simulink model "hpt_dual_hpt_sac"  (R2025a)
settings: Solver=ode23tb  StartTime=0.0  StopTime=0.6  RelTol=1e-3
libraries: spsLinearTransformerLib x6, spsThreePhaseVIMeasurementLib x4, spsUniversalBridgeLib x4, spsSeriesRLCBranchLib x3, spsThreePhaseSeriesRLCLoadLib x2, spsThreePhaseSeriesRLCBranchLib x2, spsVoltageMeasurementLib x2, spsThreePhaseSourceLib x2, spsGroundLib x1, spsCurrentMeasurementLib x1, spspowerguiLib x1
settings Model: Creator=m1391  LastModifiedBy=m1391

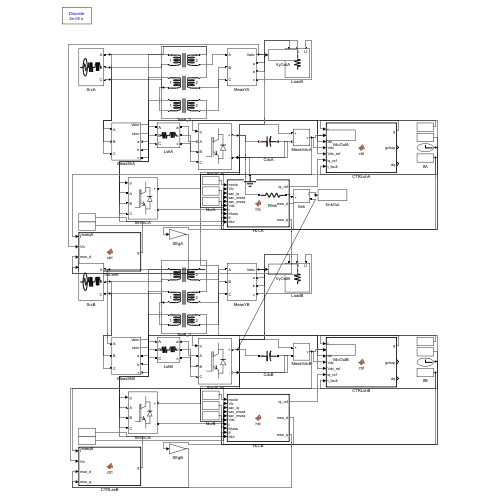
[thumbnail: Simulink's stored preview of the top-level diagram]
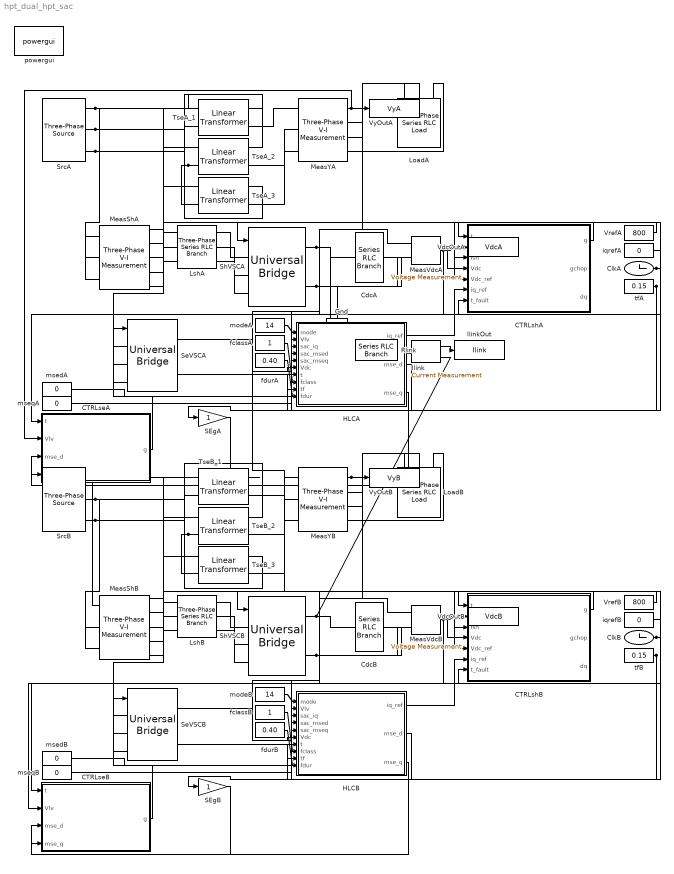
== system hpt_dual_hpt_sac ==
  CTRLseA : MATLAB Function  TreatAsAtomicUnit=on
  CTRLseB : MATLAB Function  TreatAsAtomicUnit=on
  CTRLshA : MATLAB Function  TreatAsAtomicUnit=on
  CTRLshB : MATLAB Function  TreatAsAtomicUnit=on
  CdcA : spsSeriesRLCBranchLib/Series RLC Branch  LConnTagsString=__new0  RConnTagsString=__new0  BranchType=C  Resistance=1  Inductance=1e-3  SetiL0=off  InitialCurrent=0  Capacitance=0.0022  Setx0=on  InitialVoltage=800  Measurements=None
  CdcB : spsSeriesRLCBranchLib/Series RLC Branch  LConnTagsString=__new0  RConnTagsString=__new0  BranchType=C  Resistance=1  Inductance=1e-3  SetiL0=off  InitialCurrent=0  Capacitance=0.0022  Setx0=on  InitialVoltage=800  Measurements=None
  ClkA : Clock
  ClkB : Clock
  Gnd : spsGroundLib/Ground  LConnTagsString=a
  HLCA : MATLAB Function  TreatAsAtomicUnit=on
  HLCB : MATLAB Function  TreatAsAtomicUnit=on
  Ilink : spsCurrentMeasurementLib/Current Measurement  PhasorSimulation=off  OutputType=Complex  PSBequivalent=0
  IlinkOut : ToWorkspace  VariableName=Ilink  SampleTime=2e-05
  LoadA : spsThreePhaseSeriesRLCLoadLib/Three-Phase Series RLC Load  LConnTagsString=A|B|C  Configuration=Y (floating)  NominalVoltage=400  Vabc=[1e3 1e3 1e3]  Vabcp=[1e3 1e3 1e3]  NominalFrequency=50  UnbalancedPower=off  ActivePower=400000  InductivePower=0  CapacitivePower=0  Pabc=[10e3 9e3 11e3]  QLabc=[100 90 110]  QCabc=[100 90 110]  Pabcp=[10e3 9e3 11e3]  QLabcp=[100 90 110]  QCabcp=[100 90 110]  Measurements=None  LoadType=constant Z
  LoadB : spsThreePhaseSeriesRLCLoadLib/Three-Phase Series RLC Load  LConnTagsString=A|B|C  Configuration=Y (floating)  NominalVoltage=400  Vabc=[1e3 1e3 1e3]  Vabcp=[1e3 1e3 1e3]  NominalFrequency=50  UnbalancedPower=off  ActivePower=400000  InductivePower=0  CapacitivePower=0  Pabc=[10e3 9e3 11e3]  QLabc=[100 90 110]  QCabc=[100 90 110]  Pabcp=[10e3 9e3 11e3]  QLabcp=[100 90 110]  QCabcp=[100 90 110]  Measurements=None  LoadType=constant Z
  LshA : spsThreePhaseSeriesRLCBranchLib/Three-Phase Series RLC Branch  LConnTagsString=A|B|C  RConnTagsString=A|B|C  BranchType=RL  Resistance=0.05  Inductance=0.003  Capacitance=1e-6  Measurements=None
  LshB : spsThreePhaseSeriesRLCBranchLib/Three-Phase Series RLC Branch  LConnTagsString=A|B|C  RConnTagsString=A|B|C  BranchType=RL  Resistance=0.05  Inductance=0.003  Capacitance=1e-6  Measurements=None
  MeasShA : spsThreePhaseVIMeasurementLib/Three-Phase V-I Measurement  VoltageMeasurement=phase-to-ground  SetLabelV=off  LabelV=Vabc  Vpu=off  VpuLL=off  CurrentMeasurement=yes  SetLabelI=off  LabelI=Iabc  Ipu=off  Pbase=100e6  Vbase=500e3  OutputType=Complex  PhasorSimulation=off  PSBequivalent=0
  MeasShB : spsThreePhaseVIMeasurementLib/Three-Phase V-I Measurement  VoltageMeasurement=phase-to-ground  SetLabelV=off  LabelV=Vabc  Vpu=off  VpuLL=off  CurrentMeasurement=yes  SetLabelI=off  LabelI=Iabc  Ipu=off  Pbase=100e6  Vbase=500e3  OutputType=Complex  PhasorSimulation=off  PSBequivalent=0
  MeasVdcA : spsVoltageMeasurementLib/Voltage Measurement  PhasorSimulation=off  OutputType=Complex  PSBequivalent=0
  MeasVdcB : spsVoltageMeasurementLib/Voltage Measurement  PhasorSimulation=off  OutputType=Complex  PSBequivalent=0
  MeasYA : spsThreePhaseVIMeasurementLib/Three-Phase V-I Measurement  VoltageMeasurement=phase-to-ground  SetLabelV=off  LabelV=Vabc  Vpu=off  VpuLL=off  CurrentMeasurement=no  SetLabelI=off  LabelI=Iabc  Ipu=off  Pbase=100e6  Vbase=500e3  OutputType=Complex  PhasorSimulation=off  PSBequivalent=0
  MeasYB : spsThreePhaseVIMeasurementLib/Three-Phase V-I Measurement  VoltageMeasurement=phase-to-ground  SetLabelV=off  LabelV=Vabc  Vpu=off  VpuLL=off  CurrentMeasurement=no  SetLabelI=off  LabelI=Iabc  Ipu=off  Pbase=100e6  Vbase=500e3  OutputType=Complex  PhasorSimulation=off  PSBequivalent=0
  Rlink : spsSeriesRLCBranchLib/Series RLC Branch  LConnTagsString=__new0  RConnTagsString=__new0  BranchType=R  Resistance=0.5  Inductance=1e-3  SetiL0=off  InitialCurrent=0  Capacitance=1e-6  Setx0=off  InitialVoltage=0  Measurements=None
  SEgA : Gain
  SEgB : Gain
  SeVSCA : spsUniversalBridgeLib/Universal Bridge  Arms=3  SnubberResistance=1e5  SnubberCapacitance=inf  Device=IGBT / Diodes  Ron=1e-3  Lon=0  ForwardVoltages="[  0  0  ]"  ForwardVoltage=0  GTOparameters=[ 10e-6 , 20e-6 ]  IGBTparameters=[ 1e-6 , 2e-6 ]  Measurements=None  Measurements_2=None  converterType=Rectifier
  SeVSCB : spsUniversalBridgeLib/Universal Bridge  Arms=3  SnubberResistance=1e5  SnubberCapacitance=inf  Device=IGBT / Diodes  Ron=1e-3  Lon=0  ForwardVoltages="[  0  0  ]"  ForwardVoltage=0  GTOparameters=[ 10e-6 , 20e-6 ]  IGBTparameters=[ 1e-6 , 2e-6 ]  Measurements=None  Measurements_2=None  converterType=Rectifier
  ShVSCA : spsUniversalBridgeLib/Universal Bridge  Arms=3  SnubberResistance=1e5  SnubberCapacitance=inf  Device=IGBT / Diodes  Ron=1e-3  Lon=0  ForwardVoltages="[  0  0  ]"  ForwardVoltage=0  GTOparameters=[ 10e-6 , 20e-6 ]  IGBTparameters=[ 1e-6 , 2e-6 ]  Measurements=None  Measurements_2=None  converterType=Rectifier
  ShVSCB : spsUniversalBridgeLib/Universal Bridge  Arms=3  SnubberResistance=1e5  SnubberCapacitance=inf  Device=IGBT / Diodes  Ron=1e-3  Lon=0  ForwardVoltages="[  0  0  ]"  ForwardVoltage=0  GTOparameters=[ 10e-6 , 20e-6 ]  IGBTparameters=[ 1e-6 , 2e-6 ]  Measurements=None  Measurements_2=None  converterType=Rectifier
  SrcA : spsThreePhaseSourceLib/Three-Phase Source  InternalConnection=Y  VoltagePhases=off  Voltage=400  PhaseAngle=0  Voltage_phases=[25e3 25e3 25e3]/sqrt(3)  PhaseAngles_phases=[0 -120 +120]  Frequency=50  NonIdealSource=on  SpecifyImpedance=off  Resistance=1e-3  Inductance=1e-5  ShortCircuitLevel=100e6  BaseVoltage=25e3  XRratio=7  BusType=swing  Pref=10e3  Qref=0  Prefabc=[10e3, 10e3, 10e3]  Qrefabc=[0, 0, 0]  Qmin=-inf  Qmax=inf
  SrcB : spsThreePhaseSourceLib/Three-Phase Source  InternalConnection=Y  VoltagePhases=off  Voltage=400  PhaseAngle=0  Voltage_phases=[25e3 25e3 25e3]/sqrt(3)  PhaseAngles_phases=[0 -120 +120]  Frequency=50  NonIdealSource=on  SpecifyImpedance=off  Resistance=1e-3  Inductance=1e-5  ShortCircuitLevel=100e6  BaseVoltage=25e3  XRratio=7  BusType=swing  Pref=10e3  Qref=0  Prefabc=[10e3, 10e3, 10e3]  Qrefabc=[0, 0, 0]  Qmin=-inf  Qmax=inf
  TseA_1 : spsLinearTransformerLib/Linear Transformer  UNITS=pu  NominalPower=[30000,50]  winding1=[400,0.002,0.03]  winding2=[46.2,0.002,0.03]  ThreeWindings=off  winding3=[ 315e3 0.002 0.08 ]  RmLm=[ 500 500 ]  Measurements=None  DataType=off
  TseA_2 : spsLinearTransformerLib/Linear Transformer  UNITS=pu  NominalPower=[30000,50]  winding1=[400,0.002,0.03]  winding2=[46.2,0.002,0.03]  ThreeWindings=off  winding3=[ 315e3 0.002 0.08 ]  RmLm=[ 500 500 ]  Measurements=None  DataType=off
  TseA_3 : spsLinearTransformerLib/Linear Transformer  UNITS=pu  NominalPower=[30000,50]  winding1=[400,0.002,0.03]  winding2=[46.2,0.002,0.03]  ThreeWindings=off  winding3=[ 315e3 0.002 0.08 ]  RmLm=[ 500 500 ]  Measurements=None  DataType=off
  TseB_1 : spsLinearTransformerLib/Linear Transformer  UNITS=pu  NominalPower=[30000,50]  winding1=[400,0.002,0.03]  winding2=[46.2,0.002,0.03]  ThreeWindings=off  winding3=[ 315e3 0.002 0.08 ]  RmLm=[ 500 500 ]  Measurements=None  DataType=off
  TseB_2 : spsLinearTransformerLib/Linear Transformer  UNITS=pu  NominalPower=[30000,50]  winding1=[400,0.002,0.03]  winding2=[46.2,0.002,0.03]  ThreeWindings=off  winding3=[ 315e3 0.002 0.08 ]  RmLm=[ 500 500 ]  Measurements=None  DataType=off
  TseB_3 : spsLinearTransformerLib/Linear Transformer  UNITS=pu  NominalPower=[30000,50]  winding1=[400,0.002,0.03]  winding2=[46.2,0.002,0.03]  ThreeWindings=off  winding3=[ 315e3 0.002 0.08 ]  RmLm=[ 500 500 ]  Measurements=None  DataType=off
  VdcOutA : ToWorkspace  VariableName=VdcA  SampleTime=2e-05
  VdcOutB : ToWorkspace  VariableName=VdcB  SampleTime=2e-05
  VrefA : Constant  Value=800
  VrefB : Constant  Value=800
  VyOutA : ToWorkspace  VariableName=VyA  SampleTime=2e-05
  VyOutB : ToWorkspace  VariableName=VyB  SampleTime=2e-05
  fclassA : Constant
  fclassB : Constant
  fdurA : Constant  Value=0.40
  fdurB : Constant  Value=0.40
  iqrefA : Constant  Value=0
  iqrefB : Constant  Value=0
  modeA : Constant  Value=14
  modeB : Constant  Value=14
  msedA : Constant  Value=0
  msedB : Constant  Value=0
  mseqA : Constant  Value=0
  mseqB : Constant  Value=0
  powergui : spspowerguiLib/powergui  Priority=1  SimulationMode=Discrete  SampleTime=2e-05  frequency=60  Iterations=50  frequencyindice=60  Pbase=100e6  ErrMax=1e-4  UnitsV=kV  UnitsW=MW  buscounter=0  FunctionMessages=off  echomessages=off  EnableUseOfTLC=off  CurrentSourceSwitches=off  DisableSnubberDevices=off  DisableRonSwitches=off  DisableVfSwitches=off  DisplayEquations=off  AutomaticDiscreteSolvers=off  SolverType=Tustin/Backward Euler (TBE)  Interpol=off  ExternalGateDelay=off  methode=off  Ts=100  x0status=blocks  SPID=on  SwTol=0  HookPort=off  NonlinearTolerance=1e-4  nMaxIteration=100  ContinueOnMaxIteration=off  RestoreLinks=warning  ResistiveCurrentMeasurement=off  Frange=[0:2:500]  Ylog=off  Xlog=on  ShowGrid=off  save=off  variable=ZData  structure=0  ZoomFFT=off  StartTime=0.0  cycles=1  DisplayStyle=1  fundamental=60  FreqAxis=off  MaxFrequency=1000  frequencyindicesteady=1  RmsSteady=1  display=off
  tfA : Constant  Value=0.15
  tfB : Constant  Value=0.15
  wires:
  ClkA/1 -> CTRLshA/1(t), CTRLseA/1(t), HLCA/7(t)
  MeasShA/1 -> CTRLshA/2(Vabc)
  MeasShA/2 -> CTRLshA/3(Ish)
  MeasVdcA/1 -> CTRLshA/4(Vdc), HLCA/6(Vdc), VdcOutA/1
  VrefA/1 -> CTRLshA/5(Vdc_ref)
  tfA/1 -> CTRLshA/7(t_fault), HLCA/9(tf)
  CTRLshA/1(g) -> ShVSCA/1
  MeasYA/1 -> CTRLseA/2(Vlv), HLCA/2(Vlv), VyOutA/1
  CTRLseA/1(g) -> SeVSCA/1
  modeA/1 -> HLCA/1(mode)
  iqrefA/1 -> HLCA/3(sac_iq)
  msedA/1 -> HLCA/4(sac_msed)
  mseqA/1 -> HLCA/5(sac_mseq)
  fclassA/1 -> HLCA/8(fclass)
  fdurA/1 -> HLCA/10(fdur)
  HLCA/1(iq_ref) -> CTRLshA/6(iq_ref)
  HLCA/2(mse_d) -> SEgA/1
  SEgA/1 -> CTRLseA/3(mse_d)
  HLCA/3(mse_q) -> CTRLseA/4(mse_q)
  ClkB/1 -> CTRLshB/1(t), CTRLseB/1(t), HLCB/7(t)
  MeasShB/1 -> CTRLshB/2(Vabc)
  MeasShB/2 -> CTRLshB/3(Ish)
  MeasVdcB/1 -> CTRLshB/4(Vdc), HLCB/6(Vdc), VdcOutB/1
  VrefB/1 -> CTRLshB/5(Vdc_ref)
  tfB/1 -> CTRLshB/7(t_fault), HLCB/9(tf)
  CTRLshB/1(g) -> ShVSCB/1
  MeasYB/1 -> CTRLseB/2(Vlv), HLCB/2(Vlv), VyOutB/1
  CTRLseB/1(g) -> SeVSCB/1
  modeB/1 -> HLCB/1(mode)
  iqrefB/1 -> HLCB/3(sac_iq)
  msedB/1 -> HLCB/4(sac_msed)
  mseqB/1 -> HLCB/5(sac_mseq)
  fclassB/1 -> HLCB/8(fclass)
  fdurB/1 -> HLCB/10(fdur)
  HLCB/1(iq_ref) -> CTRLshB/6(iq_ref)
  HLCB/2(mse_d) -> SEgB/1
  SEgB/1 -> CTRLseB/3(mse_d)
  HLCB/3(mse_q) -> CTRLseB/4(mse_q)
  Ilink/1 -> IlinkOut/1
  connections:
  TseA_1/RConn1 -- SrcA/RConn1 -- MeasShA/LConn1
  TseA_1/RConn2 -- MeasYA/LConn1
  MeasYA/RConn1 -- LoadA/LConn1
  MeasShA/RConn1 -- LshA/LConn1
  LshA/RConn1 -- ShVSCA/LConn1
  SeVSCA/LConn1 -- TseA_1/LConn1
  TseA_2/RConn1 -- SrcA/RConn2 -- MeasShA/LConn2
  TseA_2/RConn2 -- MeasYA/LConn2
  MeasYA/RConn2 -- LoadA/LConn2
  MeasShA/RConn2 -- LshA/LConn2
  LshA/RConn2 -- ShVSCA/LConn2
  SeVSCA/LConn2 -- TseA_2/LConn1
  TseA_3/RConn1 -- SrcA/RConn3 -- MeasShA/LConn3
  TseA_3/RConn2 -- MeasYA/LConn3
  MeasYA/RConn3 -- LoadA/LConn3
  MeasShA/RConn3 -- LshA/LConn3
  LshA/RConn3 -- ShVSCA/LConn3
  SeVSCA/LConn3 -- TseA_3/LConn1
  TseA_2/LConn2 -- TseA_1/LConn2 -- TseA_3/LConn2
  CdcA/LConn1 -- ShVSCA/RConn1 -- SeVSCA/RConn1 -- MeasVdcA/LConn1 -- Rlink/LConn1
  TseB_1/RConn1 -- SrcB/RConn1 -- MeasShB/LConn1
  TseB_1/RConn2 -- MeasYB/LConn1
  MeasYB/RConn1 -- LoadB/LConn1
  MeasShB/RConn1 -- LshB/LConn1
  LshB/RConn1 -- ShVSCB/LConn1
  SeVSCB/LConn1 -- TseB_1/LConn1
  TseB_2/RConn1 -- SrcB/RConn2 -- MeasShB/LConn2
  TseB_2/RConn2 -- MeasYB/LConn2
  MeasYB/RConn2 -- LoadB/LConn2
  MeasShB/RConn2 -- LshB/LConn2
  LshB/RConn2 -- ShVSCB/LConn2
  SeVSCB/LConn2 -- TseB_2/LConn1
  TseB_3/RConn1 -- SrcB/RConn3 -- MeasShB/LConn3
  TseB_3/RConn2 -- MeasYB/LConn3
  MeasYB/RConn3 -- LoadB/LConn3
  MeasShB/RConn3 -- LshB/LConn3
  LshB/RConn3 -- ShVSCB/LConn3
  SeVSCB/LConn3 -- TseB_3/LConn1
  TseB_2/LConn2 -- TseB_1/LConn2 -- TseB_3/LConn2
  CdcB/LConn1 -- ShVSCB/RConn1 -- SeVSCB/RConn1 -- MeasVdcB/LConn1 -- Ilink/RConn1
  CdcB/RConn1 -- SeVSCB/RConn2 -- MeasVdcB/LConn2 -- ShVSCB/RConn2 -- CdcA/RConn1 -- SeVSCA/RConn2 -- MeasVdcA/LConn2 -- ShVSCA/RConn2 -- Gnd/LConn1
  Rlink/RConn1 -- Ilink/LConn1

== matlab function hpt_dual_hpt_sac/CTRLseA ==
  data: t input; g output; Vlv input; mse_d input; mse_q input
function g = ctrl(t, Vlv, mse_d, mse_q)
%#codegen
persistent th wint tprev
if isempty(th) || t<1e-9; th=0; wint=0; tprev=0; end
dt=t-tprev; if dt<0;dt=0;end; if dt>1e-3;dt=1e-3;end; tprev=t;
w0=2*pi*50;
Va=Vlv(1); Vb=Vlv(2); Vc=Vlv(3);
Valpha=(2/3)*(Va-0.5*Vb-0.5*Vc); Vbeta=(2/3)*(sqrt(3)/2)*(Vb-Vc);
Vd= cos(th)*Valpha+sin(th)*Vbeta; Vq=-sin(th)*Valpha+cos(th)*Vbeta;
Vm=sqrt(Vd*Vd+Vq*Vq); if Vm<50;Vm=50;end
wint=wint+1500*(Vq/Vm)*dt; if wint>150;wint=150;elseif wint<-150;wint=-150;end
w=w0+90*(Vq/Vm)+wint; th=th+w*dt; th=mod(th,2*pi);
% map SAC m_se (pu of LV phase, +/-0.2) -> VSC modulation index (+/-1): K=5
md=5*mse_d; mq=5*mse_q;
ma=md*cos(th)-mq*sin(th); mb=md*cos(th-2*pi/3)-mq*sin(th-2*pi/3); mc=md*cos(th+2*pi/3)-mq*sin(th+2*pi/3);
if ma>1;ma=1;elseif ma<-1;ma=-1;end
if mb>1;mb=1;elseif mb<-1;mb=-1;end
if mc>1;mc=1;elseif mc<-1;mc=-1;end
fc=5000; carrier=2*abs(2*(fc*t-floor(fc*t+0.5)))-1;
ga=ma>=carrier; gb=mb>=carrier; gc=mc>=carrier;
g=double([ga;~ga;gb;~gb;gc;~gc]);

== matlab function hpt_dual_hpt_sac/CTRLshA ==
  data: t input; g output; Vabc input; Ish input; Vdc input; Vdc_ref input; iq_ref input; t_fault input; gchop output; dq output
function [g, gchop, dq] = ctrl(t, Vabc, Ish, Vdc, Vdc_ref, iq_ref, t_fault)
%#codegen
persistent th wint idi iqi vdi tprev en idr
if isempty(th) || t < 1e-9
    th=0; wint=0; idi=0; iqi=0; vdi=0; tprev=0; en=0; idr=0;
end
if Vdc > 620; en = 1; end
dt = t - tprev; if dt<0; dt=0; end; if dt>1e-3; dt=1e-3; end; tprev=t;
w0 = 2*pi*50; Lsh = 3e-3; Imax = 173.2;
Va=Vabc(1); Vb=Vabc(2); Vc=Vabc(3);
Valpha=(2/3)*(Va-0.5*Vb-0.5*Vc); Vbeta=(2/3)*(sqrt(3)/2)*(Vb-Vc);
Vd =  cos(th)*Valpha + sin(th)*Vbeta;
Vq = -sin(th)*Valpha + cos(th)*Vbeta;
Vm = sqrt(Vd*Vd+Vq*Vq); if Vm<100; Vm=100; end
err = Vq/Vm;
Kp_pll=90; Ki_pll=1500;
wint = wint + Ki_pll*err*dt; if wint>150; wint=150; elseif wint<-150; wint=-150; end
w = w0 + Kp_pll*err + wint; th = th + w*dt; th = mod(th,2*pi);
Ia=Ish(1); Ib=Ish(2); Ic=Ish(3);
Ialpha=(2/3)*(Ia-0.5*Ib-0.5*Ic); Ibeta=(2/3)*(sqrt(3)/2)*(Ib-Ic);
id =  cos(th)*Ialpha + sin(th)*Ibeta;
iq = -sin(th)*Ialpha + cos(th)*Ibeta;
Kpv=0.50; Kiv=8.0; ev=(Vdc_ref-Vdc)/Vdc_ref;
vdi = vdi + Kiv*ev*dt; if vdi>1; vdi=1; elseif vdi<-1; vdi=-1; end
idtgt=(Kpv*ev+vdi)*Imax; if idtgt>0.9*Imax; idtgt=0.9*Imax; elseif idtgt<-0.9*Imax; idtgt=-0.9*Imax; end
dmax=4000*dt; ds=idtgt-idr; if ds>dmax; ds=dmax; elseif ds<-dmax; ds=-dmax; end; idr=idr+ds;
iqr=iq_ref; if iqr>0.3*Imax; iqr=0.3*Imax; elseif iqr<-0.3*Imax; iqr=-0.3*Imax; end
idm=sqrt(max(0,Imax*Imax-iqr*iqr)); if idr<-idm; idr=-idm; elseif idr>idm; idr=idm; end
Kp=2.5; Ki=150; ed=idr-id; eq=iqr-iq;
ud = Vd-(Kp*ed+idi)+w0*Lsh*iq;
uq = Vq-(Kp*eq+iqi)-w0*Lsh*id;
half=max(50,Vdc/2); md=ud/half; mq=uq/half;
ma=md*cos(th)-mq*sin(th); mb=md*cos(th-2*pi/3)-mq*sin(th-2*pi/3); mc=md*cos(th+2*pi/3)-mq*sin(th+2*pi/3);
if ma>1; ma=1; elseif ma<-1; ma=-1; end
if mb>1; mb=1; elseif mb<-1; mb=-1; end
if mc>1; mc=1; elseif mc<-1; mc=-1; end
fc=5000; carrier=2*abs(2*(fc*t-floor(fc*t+0.5)))-1;
ga=ma>=carrier; gb=mb>=carrier; gc=mc>=carrier;
g=double([ga;~ga;gb;~gb;gc;~gc]);
if en<0.5; g=zeros(6,1); idi=0; iqi=0; vdi=0; end
sat=(abs(md)>1)||(abs(mq)>1);
if ~sat; idi=idi+Ki*ed*dt; iqi=iqi+Ki*eq*dt; if idi>300;idi=300;elseif idi<-300;idi=-300;end; if iqi>300;iqi=300;elseif iqi<-300;iqi=-300;end; end
gchop = double(Vdc > 1.20*800);
dq = [id; iq; idr; iqr; Vd; Vm; th];

== matlab function hpt_dual_hpt_sac/HLCA ==
  data: mode input; iq_ref output; Vlv input; sac_iq input; sac_msed input; sac_mseq input; Vdc input; t input; fclass input; tf input; fdur input; mse_d output; mse_q output
function [iq_ref, mse_d, mse_q] = hlc(mode, Vlv, sac_iq, sac_msed, sac_mseq, Vdc, t, fclass, tf, fdur)
%#codegen
% build-nonce 20260617-040759-577: forces fresh codegen so coder.load re-reads weight .mat files
persistent ba bb bi la vpf vnf kstep ahold
if isempty(ba); ba=zeros(250,1); bb=zeros(250,1); bi=1; la=zeros(4,1); vpf=1; vnf=0; kstep=int32(0); ahold=zeros(4,1); end
Imax=173.2; Vnom=326.6;
iq_ref=0; mse_d=0; mse_q=0;
Va=Vlv(1); Vb=Vlv(2); Vc=Vlv(3);
Valpha=(2/3)*(Va-0.5*Vb-0.5*Vc); Vbeta=(2/3)*(sqrt(3)/2)*(Vb-Vc);
Vpu=sqrt(Valpha*Valpha+Vbeta*Vbeta)/Vnom;
mi=int32(mode);
if mi==11 || mi==12 || mi==13 || mi==14
    % ===== closed-loop SAC (11=single, 12=gated 4-expert), 21-D obs each step =====
    NB=250;
    Vad=ba(bi); Vbd=bb(bi); ba(bi)=Valpha; bb(bi)=Vbeta; bi=bi+1; if bi>NB; bi=1; end
    V1a=0.5*(Valpha-Vbd); V1b=0.5*(Vbeta+Vad);
    V2a=0.5*(Valpha+Vbd); V2b=0.5*(Vbeta-Vad);
    V2p=sqrt(V1a*V1a+V1b*V1b)/Vnom; V2n=sqrt(V2a*V2a+V2b*V2b)/Vnom;
    af=0.005; vpf=vpf+af*(V2p-vpf); vnf=vnf+af*(V2n-vnf); V2p=vpf; V2n=vnf;
    fc=fclass;
    if mi==12 || mi==13 || mi==14
        if V2p>1.1; fc=5; elseif V2n>0.05; fc=2; else; fc=1; end
    end
    piq=0; pmb=0;
    if V2p<0.9
        piq=1.5*(0.9-V2p); if piq>0.27; piq=0.27; end
        sgi=0.08*piq/max(0.3,V2p); fb=(Vdc/800-0.80)/0.04; if fb<0; fb=0; elseif fb>1; fb=1; end
        pmb=(0.18-sgi)/1.9; if pmb<0; pmb=0; elseif pmb>0.2; pmb=0.2; end; pmb=pmb*fb;
    elseif V2p>1.1
        piq=-1.5*(V2p-1.1); if piq<-0.27; piq=-0.27; end
        pmb=-1.5*(V2p-1.1); if pmb<-0.2; pmb=-0.2; end
    end
    if mi==13 && V2p>1.1
        % hybrid mode: HVRT domain -> analytic MPC law (mode-8 logic); LVRT -> SAC experts below
        iqp13=-1.5*(V2p-1.1); if iqp13<-0.27; iqp13=-0.27; end
        iq_ref=iqp13*Imax;
        mb13=1.5*(V2p-1.1); if mb13>0.2; mb13=0.2; end
        mse_d=mb13; mse_q=0;
    else
    kstep=kstep+int32(1); if kstep>int32(100); kstep=int32(1); end
    if kstep==int32(1)
    iqp=la(2); vdev=0.9-V2p;
    if V2p<0.9; idr=1.5*(0.9-V2p); if idr>0.3; idr=0.3; end; elseif V2p>1.1; idr=-1.5*(V2p-1.1); if idr<-0.3; idr=-0.3; end; else; idr=0; end
    iqerr=idr-iqp;
    infault=double(t>=tf && t<=tf+fdur);
    probs=zeros(6,1);
    if infault>0.5; ci=round(fc)+1; if ci<1; ci=1; elseif ci>6; ci=6; end; probs(ci)=0.92; probs(1)=probs(1)+0.08; else; probs(1)=1; end
    tfrac=(t-tf)*0.2/0.5; if tfrac<0; tfrac=0; elseif tfrac>1; tfrac=1; end
    obs=reshape([Vdc/800; V2p; V2n; abs(iqp); 0; 0; vdev; iqerr; iqp; probs; tfrac; infault; la(1); la(2); la(3); la(4)],21,1);
    if mi==11
        W=coder.load('sac_actor_weights.mat');
    elseif mi==14
        W=coder.load('sac_residual_weights.mat');
    else
        if V2p>1.1
            if V2n>0.05; W=coder.load('sac_hvrt_asym_weights.mat'); else; W=coder.load('sac_hvrt_sym_weights.mat'); end
        elseif V2n>0.05; W=coder.load('sac_asym_weights.mat');
        else; W=coder.load('sac_sym_weights.mat'); end
    end
    W0=reshape(W.latent_pi_0_weight,256,21); b0=reshape(W.latent_pi_0_bias,256,1);
    W2=reshape(W.latent_pi_2_weight,256,256); b2=reshape(W.latent_pi_2_bias,256,1);
    W4=reshape(W.latent_pi_4_weight,256,256); b4=reshape(W.latent_pi_4_bias,256,1);
    Wm=reshape(W.mu_weight,4,256); bm=reshape(W.mu_bias,4,1);
    alo=reshape(W.act_low,4,1); ahi=reshape(W.act_high,4,1);
    h=max(0, W0*obs + b0); h=max(0, W2*h + b2); h=max(0, W4*h + b4);
    mu=Wm*h + bm; at=tanh(mu); act=alo + 0.5*(at+1).*(ahi-alo);
    if (mi==12 || mi==13 || mi==14) && V2p>=0.9 && V2p<=1.1 && infault<0.5; act=zeros(4,1); end
    la=act; ahold=act;
    else
    act=ahold;
    end
    if mi==14
        % residual mode: total = receding MPC prior + held residual, clipped to physical caps.
        % asym-aware iq cap (0.24): measured peak = cmd x k_2w; ODE cannot see ripple (m14-v1 lesson)
        cap14=0.27; if V2n>0.05 && V2p<0.9; cap14=0.24; end
        a2=piq+act(2); if a2>cap14; a2=cap14; elseif a2<-cap14; a2=-cap14; end
        a3=pmb+act(3); if a3>0.2; a3=0.2; elseif a3<-0.2; a3=-0.2; end
        a4=act(4); if a4>0.2; a4=0.2; elseif a4<-0.2; a4=-0.2; end
        iq_ref=a2*Imax; mse_d=-a3; mse_q=-a4;
    else
        iq_ref=act(2)*Imax; mse_d=-act(3); mse_q=-act(4);
    end
    end
elseif mi==10
    iq_ref=sac_iq; mse_d=-sac_msed; mse_q=-sac_mseq;
else
    % dq traditional variants. All share the GB/T reactive droop (K1=1.5, cap 0.3 pu):
    if Vpu<0.9; iqp=1.5*(0.9-Vpu); if iqp>0.3; iqp=0.3; end; iq_ref=iqp*Imax;
    elseif Vpu>1.1; iqp=-1.5*(Vpu-1.1); if iqp<-0.3; iqp=-0.3; end; iq_ref=iqp*Imax;
    else; iq_ref=0; end
    if mi==8
        % week3 decision-layer one-step MPC: constrained optimum on the CALIBRATED model, receding horizon @2ms.
        % max voltage support s.t. |iq|<=0.27, Vdc_eq>=0.82 (Vdc_eq = 1 - 0.08|iq|/max(0.3,V) - 1.9*boost), |mse|<=0.2.
        % Algebraic model => closed-form optimum: series boost used UP TO the DC-budget bound (vs mode5/7 zeroing).
        if iq_ref>0.27*Imax; iq_ref=0.27*Imax; elseif iq_ref<-0.27*Imax; iq_ref=-0.27*Imax; end
        iqpu=iq_ref/Imax;
        if Vpu<0.9
            sgi=0.08*abs(iqpu)/max(0.3,Vpu);
            mb=(1.0-0.82-sgi)/1.9; if mb<0; mb=0; elseif mb>0.2; mb=0.2; end
            fb=(Vdc/800-0.80)/0.04; if fb<0; fb=0; elseif fb>1; fb=1; end
            mse_d=-mb*fb; mse_q=0;
        elseif Vpu>1.1
            mb=1.5*(Vpu-1.1); if mb>0.2; mb=0.2; end
            mse_d=mb; mse_q=0;
        else
            mse_d=0; mse_q=0;
        end
    elseif mi==7
        % Song-style + RL-backported iq headroom cap (0.27): strongest fixed-law baseline
        if iq_ref>0.27*Imax; iq_ref=0.27*Imax; elseif iq_ref<-0.27*Imax; iq_ref=-0.27*Imax; end
        mse_d=0; mse_q=0;
    elseif mi==5
        % Song-style (HPT w/o storage, lit. default): NO series action during FRT
        mse_d=0; mse_q=0;
    elseif mi==6
        % Jia-style DC-budget-aware: proportional series, linearly derated as Vdc sags
        md=-0.6*(1-Vpu); if md>0.2; md=0.2; elseif md<-0.2; md=-0.2; end
        der=(Vdc/800-0.78)/(0.95-0.78); if der<0; der=0; elseif der>1; der=1; end
        mse_d=md*der; mse_q=0;
    else
        % mode 4 (legacy baseline): fixed proportional series support
        md=-0.6*(1-Vpu); if md>0.2; md=0.2; elseif md<-0.2; md=-0.2; end
        mse_d=md; mse_q=0;
    end
end

== matlab function hpt_dual_hpt_sac/CTRLshB ==
  data: t input; g output; Vabc input; Ish input; Vdc input; Vdc_ref input; iq_ref input; t_fault input; gchop output; dq output
function [g, gchop, dq] = ctrl(t, Vabc, Ish, Vdc, Vdc_ref, iq_ref, t_fault)
%#codegen
persistent th wint idi iqi vdi tprev en idr
if isempty(th) || t < 1e-9
    th=0; wint=0; idi=0; iqi=0; vdi=0; tprev=0; en=0; idr=0;
end
if Vdc > 620; en = 1; end
dt = t - tprev; if dt<0; dt=0; end; if dt>1e-3; dt=1e-3; end; tprev=t;
w0 = 2*pi*50; Lsh = 3e-3; Imax = 173.2;
Va=Vabc(1); Vb=Vabc(2); Vc=Vabc(3);
Valpha=(2/3)*(Va-0.5*Vb-0.5*Vc); Vbeta=(2/3)*(sqrt(3)/2)*(Vb-Vc);
Vd =  cos(th)*Valpha + sin(th)*Vbeta;
Vq = -sin(th)*Valpha + cos(th)*Vbeta;
Vm = sqrt(Vd*Vd+Vq*Vq); if Vm<100; Vm=100; end
err = Vq/Vm;
Kp_pll=90; Ki_pll=1500;
wint = wint + Ki_pll*err*dt; if wint>150; wint=150; elseif wint<-150; wint=-150; end
w = w0 + Kp_pll*err + wint; th = th + w*dt; th = mod(th,2*pi);
Ia=Ish(1); Ib=Ish(2); Ic=Ish(3);
Ialpha=(2/3)*(Ia-0.5*Ib-0.5*Ic); Ibeta=(2/3)*(sqrt(3)/2)*(Ib-Ic);
id =  cos(th)*Ialpha + sin(th)*Ibeta;
iq = -sin(th)*Ialpha + cos(th)*Ibeta;
Kpv=0.50; Kiv=8.0; ev=(Vdc_ref-Vdc)/Vdc_ref;
vdi = vdi + Kiv*ev*dt; if vdi>1; vdi=1; elseif vdi<-1; vdi=-1; end
idtgt=(Kpv*ev+vdi)*Imax; if idtgt>0.9*Imax; idtgt=0.9*Imax; elseif idtgt<-0.9*Imax; idtgt=-0.9*Imax; end
dmax=4000*dt; ds=idtgt-idr; if ds>dmax; ds=dmax; elseif ds<-dmax; ds=-dmax; end; idr=idr+ds;
iqr=iq_ref; if iqr>0.3*Imax; iqr=0.3*Imax; elseif iqr<-0.3*Imax; iqr=-0.3*Imax; end
idm=sqrt(max(0,Imax*Imax-iqr*iqr)); if idr<-idm; idr=-idm; elseif idr>idm; idr=idm; end
Kp=2.5; Ki=150; ed=idr-id; eq=iqr-iq;
ud = Vd-(Kp*ed+idi)+w0*Lsh*iq;
uq = Vq-(Kp*eq+iqi)-w0*Lsh*id;
half=max(50,Vdc/2); md=ud/half; mq=uq/half;
ma=md*cos(th)-mq*sin(th); mb=md*cos(th-2*pi/3)-mq*sin(th-2*pi/3); mc=md*cos(th+2*pi/3)-mq*sin(th+2*pi/3);
if ma>1; ma=1; elseif ma<-1; ma=-1; end
if mb>1; mb=1; elseif mb<-1; mb=-1; end
if mc>1; mc=1; elseif mc<-1; mc=-1; end
fc=5000; carrier=2*abs(2*(fc*t-floor(fc*t+0.5)))-1;
ga=ma>=carrier; gb=mb>=carrier; gc=mc>=carrier;
g=double([ga;~ga;gb;~gb;gc;~gc]);
if en<0.5; g=zeros(6,1); idi=0; iqi=0; vdi=0; end
sat=(abs(md)>1)||(abs(mq)>1);
if ~sat; idi=idi+Ki*ed*dt; iqi=iqi+Ki*eq*dt; if idi>300;idi=300;elseif idi<-300;idi=-300;end; if iqi>300;iqi=300;elseif iqi<-300;iqi=-300;end; end
gchop = double(Vdc > 1.20*800);
dq = [id; iq; idr; iqr; Vd; Vm; th];

== matlab function hpt_dual_hpt_sac/CTRLseB ==
  data: t input; g output; Vlv input; mse_d input; mse_q input
function g = ctrl(t, Vlv, mse_d, mse_q)
%#codegen
persistent th wint tprev
if isempty(th) || t<1e-9; th=0; wint=0; tprev=0; end
dt=t-tprev; if dt<0;dt=0;end; if dt>1e-3;dt=1e-3;end; tprev=t;
w0=2*pi*50;
Va=Vlv(1); Vb=Vlv(2); Vc=Vlv(3);
Valpha=(2/3)*(Va-0.5*Vb-0.5*Vc); Vbeta=(2/3)*(sqrt(3)/2)*(Vb-Vc);
Vd= cos(th)*Valpha+sin(th)*Vbeta; Vq=-sin(th)*Valpha+cos(th)*Vbeta;
Vm=sqrt(Vd*Vd+Vq*Vq); if Vm<50;Vm=50;end
wint=wint+1500*(Vq/Vm)*dt; if wint>150;wint=150;elseif wint<-150;wint=-150;end
w=w0+90*(Vq/Vm)+wint; th=th+w*dt; th=mod(th,2*pi);
% map SAC m_se (pu of LV phase, +/-0.2) -> VSC modulation index (+/-1): K=5
md=5*mse_d; mq=5*mse_q;
ma=md*cos(th)-mq*sin(th); mb=md*cos(th-2*pi/3)-mq*sin(th-2*pi/3); mc=md*cos(th+2*pi/3)-mq*sin(th+2*pi/3);
if ma>1;ma=1;elseif ma<-1;ma=-1;end
if mb>1;mb=1;elseif mb<-1;mb=-1;end
if mc>1;mc=1;elseif mc<-1;mc=-1;end
fc=5000; carrier=2*abs(2*(fc*t-floor(fc*t+0.5)))-1;
ga=ma>=carrier; gb=mb>=carrier; gc=mc>=carrier;
g=double([ga;~ga;gb;~gb;gc;~gc]);

== matlab function hpt_dual_hpt_sac/HLCB ==
  data: mode input; iq_ref output; Vlv input; sac_iq input; sac_msed input; sac_mseq input; Vdc input; t input; fclass input; tf input; fdur input; mse_d output; mse_q output
function [iq_ref, mse_d, mse_q] = hlc(mode, Vlv, sac_iq, sac_msed, sac_mseq, Vdc, t, fclass, tf, fdur)
%#codegen
% build-nonce 20260617-040801-384: forces fresh codegen so coder.load re-reads weight .mat files
persistent ba bb bi la vpf vnf kstep ahold
if isempty(ba); ba=zeros(250,1); bb=zeros(250,1); bi=1; la=zeros(4,1); vpf=1; vnf=0; kstep=int32(0); ahold=zeros(4,1); end
Imax=173.2; Vnom=326.6;
iq_ref=0; mse_d=0; mse_q=0;
Va=Vlv(1); Vb=Vlv(2); Vc=Vlv(3);
Valpha=(2/3)*(Va-0.5*Vb-0.5*Vc); Vbeta=(2/3)*(sqrt(3)/2)*(Vb-Vc);
Vpu=sqrt(Valpha*Valpha+Vbeta*Vbeta)/Vnom;
mi=int32(mode);
if mi==11 || mi==12 || mi==13 || mi==14
    % ===== closed-loop SAC (11=single, 12=gated 4-expert), 21-D obs each step =====
    NB=250;
    Vad=ba(bi); Vbd=bb(bi); ba(bi)=Valpha; bb(bi)=Vbeta; bi=bi+1; if bi>NB; bi=1; end
    V1a=0.5*(Valpha-Vbd); V1b=0.5*(Vbeta+Vad);
    V2a=0.5*(Valpha+Vbd); V2b=0.5*(Vbeta-Vad);
    V2p=sqrt(V1a*V1a+V1b*V1b)/Vnom; V2n=sqrt(V2a*V2a+V2b*V2b)/Vnom;
    af=0.005; vpf=vpf+af*(V2p-vpf); vnf=vnf+af*(V2n-vnf); V2p=vpf; V2n=vnf;
    fc=fclass;
    if mi==12 || mi==13 || mi==14
        if V2p>1.1; fc=5; elseif V2n>0.05; fc=2; else; fc=1; end
    end
    piq=0; pmb=0;
    if V2p<0.9
        piq=1.5*(0.9-V2p); if piq>0.27; piq=0.27; end
        sgi=0.08*piq/max(0.3,V2p); fb=(Vdc/800-0.80)/0.04; if fb<0; fb=0; elseif fb>1; fb=1; end
        pmb=(0.18-sgi)/1.9; if pmb<0; pmb=0; elseif pmb>0.2; pmb=0.2; end; pmb=pmb*fb;
    elseif V2p>1.1
        piq=-1.5*(V2p-1.1); if piq<-0.27; piq=-0.27; end
        pmb=-1.5*(V2p-1.1); if pmb<-0.2; pmb=-0.2; end
    end
    if mi==13 && V2p>1.1
        % hybrid mode: HVRT domain -> analytic MPC law (mode-8 logic); LVRT -> SAC experts below
        iqp13=-1.5*(V2p-1.1); if iqp13<-0.27; iqp13=-0.27; end
        iq_ref=iqp13*Imax;
        mb13=1.5*(V2p-1.1); if mb13>0.2; mb13=0.2; end
        mse_d=mb13; mse_q=0;
    else
    kstep=kstep+int32(1); if kstep>int32(100); kstep=int32(1); end
    if kstep==int32(1)
    iqp=la(2); vdev=0.9-V2p;
    if V2p<0.9; idr=1.5*(0.9-V2p); if idr>0.3; idr=0.3; end; elseif V2p>1.1; idr=-1.5*(V2p-1.1); if idr<-0.3; idr=-0.3; end; else; idr=0; end
    iqerr=idr-iqp;
    infault=double(t>=tf && t<=tf+fdur);
    probs=zeros(6,1);
    if infault>0.5; ci=round(fc)+1; if ci<1; ci=1; elseif ci>6; ci=6; end; probs(ci)=0.92; probs(1)=probs(1)+0.08; else; probs(1)=1; end
    tfrac=(t-tf)*0.2/0.5; if tfrac<0; tfrac=0; elseif tfrac>1; tfrac=1; end
    obs=reshape([Vdc/800; V2p; V2n; abs(iqp); 0; 0; vdev; iqerr; iqp; probs; tfrac; infault; la(1); la(2); la(3); la(4)],21,1);
    if mi==11
        W=coder.load('sac_actor_weights.mat');
    elseif mi==14
        W=coder.load('sac_residual_weights.mat');
    else
        if V2p>1.1
            if V2n>0.05; W=coder.load('sac_hvrt_asym_weights.mat'); else; W=coder.load('sac_hvrt_sym_weights.mat'); end
        elseif V2n>0.05; W=coder.load('sac_asym_weights.mat');
        else; W=coder.load('sac_sym_weights.mat'); end
    end
    W0=reshape(W.latent_pi_0_weight,256,21); b0=reshape(W.latent_pi_0_bias,256,1);
    W2=reshape(W.latent_pi_2_weight,256,256); b2=reshape(W.latent_pi_2_bias,256,1);
    W4=reshape(W.latent_pi_4_weight,256,256); b4=reshape(W.latent_pi_4_bias,256,1);
    Wm=reshape(W.mu_weight,4,256); bm=reshape(W.mu_bias,4,1);
    alo=reshape(W.act_low,4,1); ahi=reshape(W.act_high,4,1);
    h=max(0, W0*obs + b0); h=max(0, W2*h + b2); h=max(0, W4*h + b4);
    mu=Wm*h + bm; at=tanh(mu); act=alo + 0.5*(at+1).*(ahi-alo);
    if (mi==12 || mi==13 || mi==14) && V2p>=0.9 && V2p<=1.1 && infault<0.5; act=zeros(4,1); end
    la=act; ahold=act;
    else
    act=ahold;
    end
    if mi==14
        % residual mode: total = receding MPC prior + held residual, clipped to physical caps.
        % asym-aware iq cap (0.24): measured peak = cmd x k_2w; ODE cannot see ripple (m14-v1 lesson)
        cap14=0.27; if V2n>0.05 && V2p<0.9; cap14=0.24; end
        a2=piq+act(2); if a2>cap14; a2=cap14; elseif a2<-cap14; a2=-cap14; end
        a3=pmb+act(3); if a3>0.2; a3=0.2; elseif a3<-0.2; a3=-0.2; end
        a4=act(4); if a4>0.2; a4=0.2; elseif a4<-0.2; a4=-0.2; end
        iq_ref=a2*Imax; mse_d=-a3; mse_q=-a4;
    else
        iq_ref=act(2)*Imax; mse_d=-act(3); mse_q=-act(4);
    end
    end
elseif mi==10
    iq_ref=sac_iq; mse_d=-sac_msed; mse_q=-sac_mseq;
else
    % dq traditional variants. All share the GB/T reactive droop (K1=1.5, cap 0.3 pu):
    if Vpu<0.9; iqp=1.5*(0.9-Vpu); if iqp>0.3; iqp=0.3; end; iq_ref=iqp*Imax;
    elseif Vpu>1.1; iqp=-1.5*(Vpu-1.1); if iqp<-0.3; iqp=-0.3; end; iq_ref=iqp*Imax;
    else; iq_ref=0; end
    if mi==8
        % week3 decision-layer one-step MPC: constrained optimum on the CALIBRATED model, receding horizon @2ms.
        % max voltage support s.t. |iq|<=0.27, Vdc_eq>=0.82 (Vdc_eq = 1 - 0.08|iq|/max(0.3,V) - 1.9*boost), |mse|<=0.2.
        % Algebraic model => closed-form optimum: series boost used UP TO the DC-budget bound (vs mode5/7 zeroing).
        if iq_ref>0.27*Imax; iq_ref=0.27*Imax; elseif iq_ref<-0.27*Imax; iq_ref=-0.27*Imax; end
        iqpu=iq_ref/Imax;
        if Vpu<0.9
            sgi=0.08*abs(iqpu)/max(0.3,Vpu);
            mb=(1.0-0.82-sgi)/1.9; if mb<0; mb=0; elseif mb>0.2; mb=0.2; end
            fb=(Vdc/800-0.80)/0.04; if fb<0; fb=0; elseif fb>1; fb=1; end
            mse_d=-mb*fb; mse_q=0;
        elseif Vpu>1.1
            mb=1.5*(Vpu-1.1); if mb>0.2; mb=0.2; end
            mse_d=mb; mse_q=0;
        else
            mse_d=0; mse_q=0;
        end
    elseif mi==7
        % Song-style + RL-backported iq headroom cap (0.27): strongest fixed-law baseline
        if iq_ref>0.27*Imax; iq_ref=0.27*Imax; elseif iq_ref<-0.27*Imax; iq_ref=-0.27*Imax; end
        mse_d=0; mse_q=0;
    elseif mi==5
        % Song-style (HPT w/o storage, lit. default): NO series action during FRT
        mse_d=0; mse_q=0;
    elseif mi==6
        % Jia-style DC-budget-aware: proportional series, linearly derated as Vdc sags
        md=-0.6*(1-Vpu); if md>0.2; md=0.2; elseif md<-0.2; md=-0.2; end
        der=(Vdc/800-0.78)/(0.95-0.78); if der<0; der=0; elseif der>1; der=1; end
        mse_d=md*der; mse_q=0;
    else
        % mode 4 (legacy baseline): fixed proportional series support
        md=-0.6*(1-Vpu); if md>0.2; md=0.2; elseif md<-0.2; md=-0.2; end
        mse_d=md; mse_q=0;
    end
end
